simulink model "regulator"  (R2022a)
settings: Solver=VariableStepAuto  StartTime=0.0  StopTime=50  RelTol=1e-3
values from neighbouring files (symbols this model uses):
  k1 = -3*sb - 33    (= -32.4)    [dane.m]
  k2 = 3*sb^2 -362    (= -361.88)    [dane.m]
  k3 = -sb^3 -1320    (= -1319.992)    [dane.m]
settings Model: Creator=danie  LastModifiedBy=danie

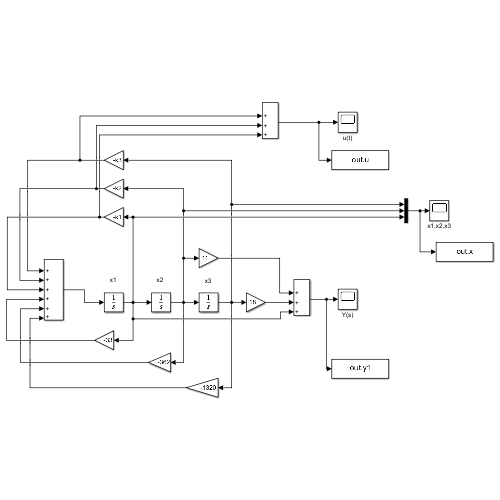
[thumbnail: Simulink's stored preview of the top-level diagram]
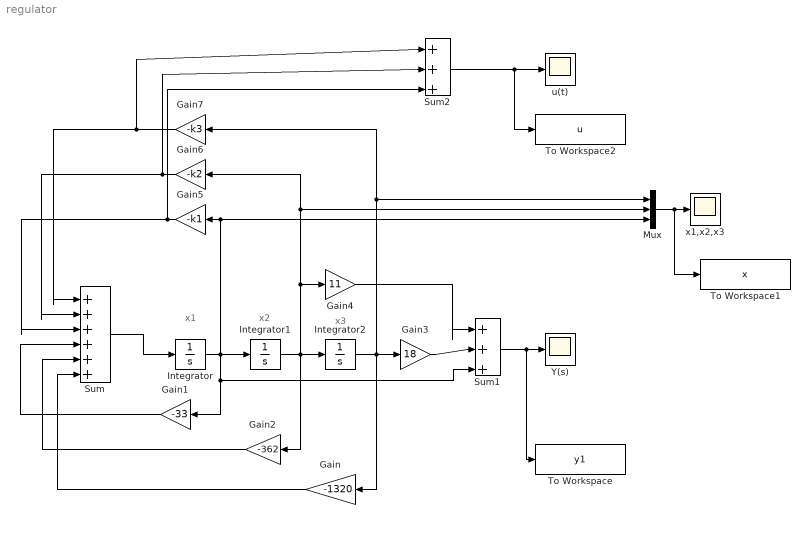
== system regulator ==
  note: x3
  note: x2
  note: x1
  Gain : Gain  Gain=-1320
  Gain1 : Gain  Gain=-33
  Gain2 : Gain  Gain=-362
  Gain3 : Gain  Gain=18
  Gain4 : Gain  Gain=11
  Gain5 : Gain  Gain=-k1
  Gain6 : Gain  Gain=-k2
  Gain7 : Gain  Gain=-k3
  Integrator : Integrator  InitialCondition=3
  Integrator1 : Integrator  InitialCondition=2
  Integrator2 : Integrator  InitialCondition=-3
  Mux : Mux  Inputs=3
  Sum : Sum  Inputs=|++++++
  Sum1 : Sum  Inputs=|+++
  Sum2 : Sum  Inputs=|+++
  To Workspace : ToWorkspace  VariableName=y1  SaveFormat=Structure With Time  SampleTime=-1
  To Workspace1 : ToWorkspace  VariableName=x  SaveFormat=Structure With Time  SampleTime=-1
  To Workspace2 : ToWorkspace  VariableName=u  SaveFormat=Structure With Time  SampleTime=-1
  Y(s) : Scope
  u(t) : Scope
  x1,x2,x3 : Scope
  wires:
  Integrator2/1 -> Gain7/1, Mux/1, Gain/1, Gain3/1
  Integrator1/1 -> Gain4/1, Gain6/1, Mux/2, Gain2/1, Integrator2/1
  Gain4/1 -> Sum1/1
  Gain2/1 -> Sum/5
  Gain/1 -> Sum/6
  Gain3/1 -> Sum1/2
  Sum1/1 -> To Workspace/1, Y(s)/1
  Sum/1 -> Integrator/1
  Gain1/1 -> Sum/4
  Integrator/1 -> Sum1/3, Gain1/1, Integrator1/1, Mux/3, Gain5/1
  Gain5/1 -> Sum2/3, Sum/3
  Gain6/1 -> Sum2/2, Sum/2
  Gain7/1 -> Sum2/1, Sum/1
  Sum2/1 -> To Workspace2/1, u(t)/1
  Mux/1 -> To Workspace1/1, x1,x2,x3/1
